simulink subsystem "env_modelling"  (R2024a)
settings: Solver=VariableStepAuto  StartTime=0.0  StopTime=10.0  RelTol=1e-3
undefined symbols (not defined in the file or in its folder): IAU, WMM2020
libraries: aerolibutil x3, aerolibtransform2 x2, matrix_library x1, vrlib x1, aerolibgravity2 x1
settings Model: Creator=joshu  LastModifiedBy=joshu

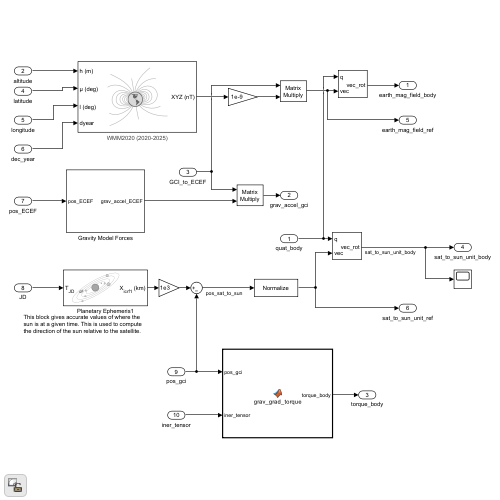
[thumbnail: Simulink's stored preview of the top-level diagram]
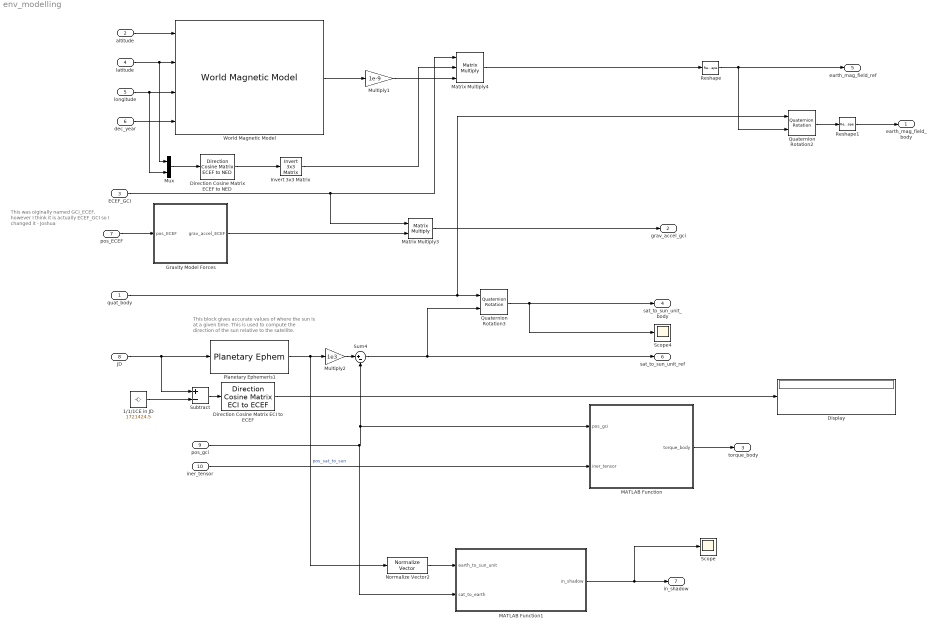
== system env_modelling ==
  note: This was oiginally named GCI_ECEF,
      | however I think it is actually ECEF_GCI
      | so I changed it
      |  - Joshua
  note: This block gives accurate values of where the sun is at a given time. This is used to compute the direction of the sun relative to the satellite.
  quat_body : Inport
  altitude : Inport  Port=2
  ECEF_GCI : Inport  Port=3
  latitude : Inport  Port=4
  longitude : Inport  Port=5
  dec_year : Inport  Port=6
  pos_ECEF : Inport  Port=7
  JD : Inport  Port=8
  pos_gci : Inport  Port=9
  iner_tensor : Inport  Port=10
  1/1/1CE in JD : Constant  Value=1721424.5
  Direction Cosine Matrix ECEF to NED : aerolibtransform2/Direction Cosine Matrix ECEF to NED
  Direction Cosine Matrix ECI to ECEF : aerolibtransform2/Direction Cosine Matrix ECI to ECEF  red=IAU-2000/2006  year=1  month=January  day=1  hour=0  min=0  sec=0  deltaT=Day  errorflag=Error  extraparamflag=off
      settings: AttributesFormatString=%<red>
  Display : Display
  Gravity Model Forces : Subsystem
  Invert 3x3 Matrix : aerolibutil/Invert  3x3 Matrix
  MATLAB Function : MATLAB Function  TreatAsAtomicUnit=on
  MATLAB Function1 : MATLAB Function  TreatAsAtomicUnit=on
  Matrix Multiply3 : Product  Multiplication=Matrix(*)
  Matrix Multiply4 : Product  Inputs=3  Multiplication=Matrix(*)
  Multiply1 : Gain  Gain=1e-9
  Multiply2 : Gain  Gain=1e3
  Mux : Mux  Inputs=2
  Normalize Vector2 : vrlib/Utilities/Normalize Vector  maxzero=0
  Planetary Ephemeris1 : PlanetaryEphem  target=Sun  outputVelocity=off
  Quaternion Rotation2 : aerolibutil/Quaternion Rotation
  Quaternion Rotation3 : aerolibutil/Quaternion Rotation
  Reshape : Reshape  OutputDimensionality=Row vector (2-D)
  Reshape1 : Reshape  OutputDimensionality=Row vector (2-D)
  Scope : Scope
  Scope4 : Scope
  Subtract : Sum  Inputs=+-
  Sum4 : Sum  Inputs=|+-
  World Magnetic Model : aerolibgravity2/World Magnetic Model  model=WMM2020 (2020-2025)  customFile='WMM2020.COF'  units=Metric (MKS)  time_in=on  month=January  day=1  year=2020  action=Warning  h_out=off  dec_out=off  inc_out=off  ti_out=off
  earth_mag_field_body : Outport  PortDimensions=[1 3]
  grav_accel_gci : Outport  Port=2
  torque_body : Outport  Port=3
  sat_to_sun_unit_body : Outport  Port=4
  earth_mag_field_ref : Outport  Port=5
  sat_to_sun_unit_ref : Outport  Port=6
  in_shadow : Outport  Port=7
  wires:
  Sum4/1 -> sat_to_sun_unit_ref/1, Quaternion Rotation3/2
  dec_year/1 -> World Magnetic Model/4
  MATLAB Function/1(torque_body) -> torque_body/1
  pos_ECEF/1 -> Gravity Model Forces/1(pos_ECEF)
  World Magnetic Model/1 -> Multiply1/1
  Matrix Multiply3/1 -> grav_accel_gci/1
  Multiply2/1 -> Sum4/1
  Quaternion Rotation3/1 -> sat_to_sun_unit_body/1, Scope4/1
  altitude/1 -> World Magnetic Model/1
  JD/1 -> Planetary Ephemeris1/1, Subtract/1
  pos_gci/1 -> Sum4/2, MATLAB Function/1(pos_gci), MATLAB Function1/2(sat_to_earth)
  Gravity Model Forces/1(grav_accel_ECEF) -> Matrix Multiply3/2
  longitude/1 -> World Magnetic Model/3, Mux/2
  ECEF_GCI/1 -> Matrix Multiply4/1, Matrix Multiply3/1
  Multiply1/1 -> Matrix Multiply4/3
  latitude/1 -> Mux/1, World Magnetic Model/2
  iner_tensor/1 -> MATLAB Function/2(iner_tensor)
  quat_body/1 -> Quaternion Rotation3/1, Quaternion Rotation2/1
  Quaternion Rotation2/1 -> Reshape1/1
  Planetary Ephemeris1/1 -> Multiply2/1, Normalize Vector2/1  "pos_sat_to_sun"
  Matrix Multiply4/1 -> Reshape/1
  1/1/1CE in JD/1 -> Subtract/2
  Subtract/1 -> Direction Cosine Matrix ECI to ECEF/1
  Direction Cosine Matrix ECI to ECEF/1 -> Display/1
  Reshape/1 -> earth_mag_field_ref/1, Quaternion Rotation2/2
  Direction Cosine Matrix ECEF to NED/1 -> Invert 3x3 Matrix/1
  Mux/1 -> Direction Cosine Matrix ECEF to NED/1
  Invert 3x3 Matrix/1 -> Matrix Multiply4/2
  Normalize Vector2/1 -> MATLAB Function1/1(earth_to_sun_unit)
  MATLAB Function1/1(in_shadow) -> in_shadow/1, Scope/1
  Reshape1/1 -> earth_mag_field_body/1

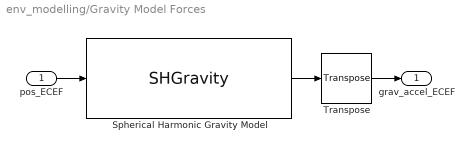
== system env_modelling/Gravity Model Forces ==
  pos_ECEF : Inport
  Spherical Harmonic Gravity Model : SHGravity
  Transpose : matrix_library/Transpose
  grav_accel_ECEF : Outport
  wires:
  pos_ECEF/1 -> Spherical Harmonic Gravity Model/1
  Transpose/1 -> grav_accel_ECEF/1
  Spherical Harmonic Gravity Model/1 -> Transpose/1

== matlab function env_modelling/MATLAB Function ==
  data: pos_gci input; torque_body output; iner_tensor input
function torque_body  = grav_grad_torque(pos_gci, iner_tensor)
    % mass of earth, grav constant
    m_e = 5.97219e24;
    G = 6.67430e-11;

    % grav param
    u = G*m_e;

    radius = norm(pos_gci);
    nadir_vec = -normalize(pos_gci);
    torque_body = cross(3*u/radius^3*nadir_vec, ...
        iner_tensor*nadir_vec);

== matlab function env_modelling/MATLAB Function1 ==
  data: earth_to_sun_unit input; in_shadow output; sat_to_earth input
function in_shadow = is_in_shadow_(earth_to_sun_unit,sat_to_earth)

in_shadow = is_in_shadow(earth_to_sun_unit,sat_to_earth);
